simulink model "SistEqLTI_aumentado"  (R2023b)
settings: Solver=VariableStepAuto  StartTime=0.0  StopTime=1  MaxStep=0.0001  RelTol=1e-3
values from neighbouring files (symbols this model uses):
  b_eq = b_m + b_l/(r^2)    (= 2.19444444444e-05)    [Parametros.m]
  C_ts = 0.818    [Parametros.m]
  g = 9.80665    [Parametros.m]
  J_eq = J_m + J_l/(r^2)    [Parametros.m]
  k_l = m*l_cm + m_l(1)*l_l    [Parametros.m]
  L_d = 6.6E-3    (= 0.0066)    [Parametros.m]
  L_q = 5.8E-3    (= 0.0058)    [Parametros.m]
  lambda_m = 0.016    [Parametros.m]
  P_p = 3    [Parametros.m]
  r = 120    [Parametros.m]
  R_tsamb = 146.7    [Parametros.m]
undefined symbols (not defined in the file or in its folder): I_d0, Rs_ref
settings Model: Creator=Tomas  LastModifiedBy=matia
settings DebuggingCC: UnconnectedInputMsg=warning  UnconnectedOutputMsg=warning  UnconnectedLineMsg=warning
settings ModelReferenceCC: EnableRefExpFcnMdlSchedulingChecks=on
settings RTWCC: DLArmComputeVersion=19.05

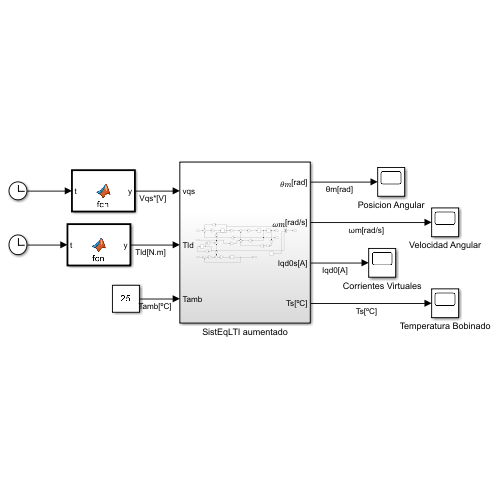
[thumbnail: Simulink's stored preview of the top-level diagram]
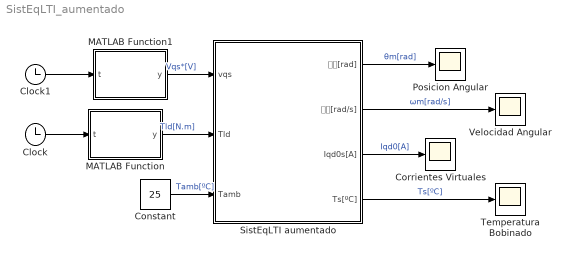
== system SistEqLTI_aumentado ==
  Clock : Clock
  Clock1 : Clock
  Constant : Constant  Value=25
  Corrientes Virtuales : Scope
  MATLAB Function : MATLAB Function  TreatAsAtomicUnit=on
  MATLAB Function1 : MATLAB Function  TreatAsAtomicUnit=on
  Posicion Angular : Scope
  SistEqLTI aumentado : Subsystem
  Temperatura Bobinado : Scope
  Velocidad Angular : Scope
  wires:
  MATLAB Function1/1(y) -> SistEqLTI aumentado/1(vqs)  "Vqs*[V]"
  MATLAB Function/1(y) -> SistEqLTI aumentado/2(Tld)  "Tld[N.m]"
  Constant/1 -> SistEqLTI aumentado/3(Tamb)  "Tamb[ºC]"
  SistEqLTI aumentado/1(𝜃𝑚[rad]) -> Posicion Angular/1  "θm[rad]"
  SistEqLTI aumentado/2(𝜔𝑚[rad/s]) -> Velocidad Angular/1  "ωm[rad/s]"
  SistEqLTI aumentado/3(Iqd0s[A]) -> Corrientes Virtuales/1  "Iqd0[A]"
  SistEqLTI aumentado/4(Ts[ºC]) -> Temperatura Bobinado/1  "Ts[ºC]"
  Clock/1 -> MATLAB Function/1(t)
  Clock1/1 -> MATLAB Function1/1(t)

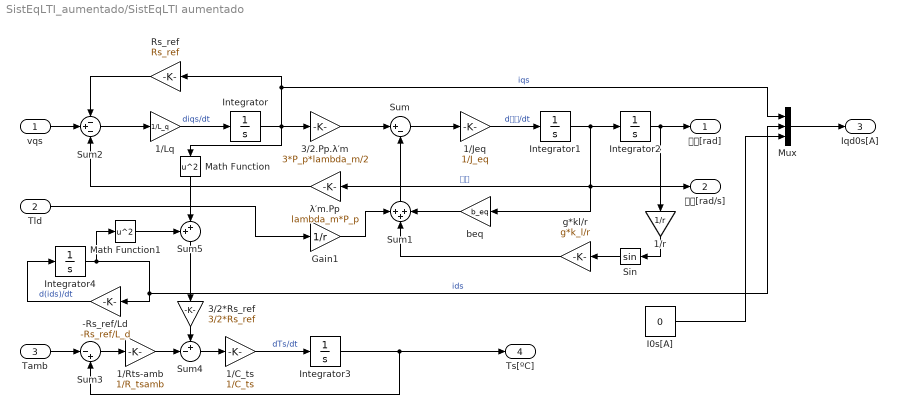
== system SistEqLTI_aumentado/SistEqLTI aumentado ==
  vqs : Inport
  Tld : Inport  Port=2
  Tamb : Inport  Port=3
  -Rs_ref/Ld : Gain  Gain=-Rs_ref/L_d
  1/C_ts : Gain  Gain=1/C_ts
  1/Jeq : Gain  Gain=1/J_eq
  1/Lq : Gain  Gain=1/L_q
  1/Rts-amb : Gain  Gain=1/R_tsamb
  1/r : Gain  Gain=1/r
  3/2*Rs_ref : Gain  Gain=3/2*Rs_ref
  3/2.Pp.λ′m : Gain  Gain=3*P_p*lambda_m/2
  Gain1 : Gain  Gain=1/r
  I0s[A] : Constant  Value=0
  Integrator{,1..3} (4 alike) : Integrator
  Integrator4 : Integrator  InitialCondition=I_d0
  Math Function : Math  Operator=square
  Math Function1 : Math  Operator=square
  Mux : Mux  Inputs=3
  Rs_ref : Gain  Gain=Rs_ref
  Sin : Trigonometry
  Sum : Sum  Inputs=|+-
  Sum1 : Sum  Inputs=+++
  Sum2 : Sum  Inputs=-+-
  Sum3 : Sum  Inputs=|-+
  Sum4 : Sum  Inputs=+-|
  Sum5 : Sum  Inputs=++|
  beq : Gain  Gain=b_eq
  g*kl/r : Gain  Gain=g*k_l/r
  λ′m.Pp : Gain  Gain=lambda_m*P_p
  𝜃𝑚[rad] : Outport
  𝜔𝑚[rad/s] : Outport  Port=2
  Iqd0s[A] : Outport  Port=3
  Ts[ºC] : Outport  Port=4
  wires:
  Tamb/1 -> Sum3/1
  Rs_ref/1 -> Sum2/1
  Integrator1/1 -> Integrator2/1, 𝜔𝑚[rad/s]/1, λ′m.Pp/1, beq/1  "𝜔𝑚"
  Sum3/1 -> 1/Rts-amb/1
  Integrator2/1 -> 𝜃𝑚[rad]/1, 1/r/1
  Integrator/1 -> 3/2.Pp.λ′m/1, Math Function/1, Rs_ref/1, Mux/1  "iqs"
  1/C_ts/1 -> Integrator3/1  "dTs/dt"
  Sum1/1 -> Sum/2
  Integrator3/1 -> Ts[ºC]/1, Sum3/2
  Sum2/1 -> 1/Lq/1
  Sum/1 -> 1/Jeq/1
  1/Lq/1 -> Integrator/1  "diqs/dt"
  3/2.Pp.λ′m/1 -> Sum/1
  Sum4/1 -> 1/C_ts/1
  1/Jeq/1 -> Integrator1/1  "d𝜔𝑚/dt"
  3/2*Rs_ref/1 -> Sum4/1
  λ′m.Pp/1 -> Sum2/3
  1/Rts-amb/1 -> Sum4/2
  Tld/1 -> Gain1/1
  beq/1 -> Sum1/3
  Gain1/1 -> Sum1/1
  Sum5/1 -> 3/2*Rs_ref/1
  g*kl/r/1 -> Sum1/2
  Integrator4/1 -> Math Function1/1, Mux/2, -Rs_ref/Ld/1  "ids"
  Sin/1 -> g*kl/r/1
  1/r/1 -> Sin/1
  vqs/1 -> Sum2/2
  Math Function1/1 -> Sum5/1
  Math Function/1 -> Sum5/2
  -Rs_ref/Ld/1 -> Integrator4/1  "d(ids)/dt"
  I0s[A]/1 -> Mux/3
  Mux/1 -> Iqd0s[A]/1

== matlab function SistEqLTI_aumentado/MATLAB Function ==
  data: t input; y output
function y = fcn(t)
    % Initialize output
    y = 0;
    
    % Generate the square signal based on time conditions
    if t >= 0.3 && t < 0.5
        y = 6.28;
    elseif t >= 0.5 && t < 0.9
        y = -6.28;
    else
        y = 0;
    end
end

== matlab function SistEqLTI_aumentado/MATLAB Function1 ==
  data: t input; y output
function y = fcn(t)
    % Initialize output
    y = 0;
    
    % Generate the square signal based on time conditions
    if t >= 0.1 && t < 0.7
        y = 19.596;
    else
        y = 0;
    end
end
